simulink model "exam_task_diffuri"  (R2021a)
settings: Solver=VariableStepAuto  StartTime=0.0  StopTime=5  RelTol=1e-3
libraries: simulink x1
settings Model: Creator=Егор  LastModifiedBy=Егор

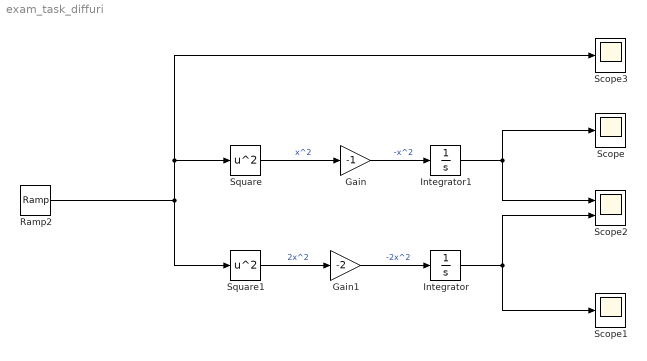
== system exam_task_diffuri ==
  Gain : Gain  Gain=-1
  Gain1 : Gain  Gain=-2
  Integrator : Integrator
  Integrator1 : Integrator
  Ramp2 : simulink/Sources/Ramp  slope=1  start=0  InitialOutput=0
  Scope : Scope
  Scope1 : Scope
  Scope2 : Scope  NumInputPorts=2
  Scope3 : Scope
  Square : Math  Operator=square  SaturateOnIntegerOverflow=on
  Square1 : Math  Operator=square  SaturateOnIntegerOverflow=on
  wires:
  Square/1 -> Gain/1  "x^2"
  Square1/1 -> Gain1/1  "2x^2"
  Integrator1/1 -> Scope2/1, Scope/1
  Integrator/1 -> Scope2/2, Scope1/1
  Gain/1 -> Integrator1/1  "-x^2"
  Gain1/1 -> Integrator/1  "-2x^2"
  Ramp2/1 -> Square1/1, Scope3/1, Square/1
